simulink model "ParmTests"  (Simulink 7.5)
settings: Solver=ode45  StartTime=0.0  StopTime=10.0  RelTol=1e-3
settings Model: Creator=Robert  LastModifiedBy=Robert

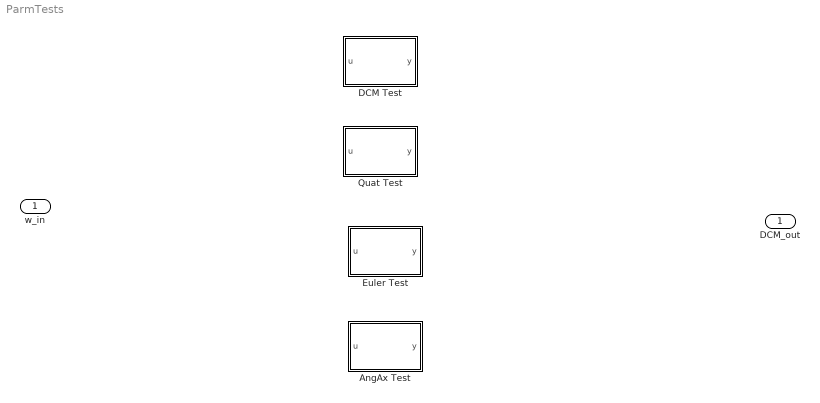
== system ParmTests ==
  w_in : Inport  OutDataType=fixdt(1, 16)  OutScaling=2^0
  AngAx Test : Stateflow chart  TreatAsAtomicUnit=on
  DCM Test : Stateflow chart  TreatAsAtomicUnit=on
  Euler Test : Stateflow chart  TreatAsAtomicUnit=on
  Quat Test : Stateflow chart  TreatAsAtomicUnit=on
  DCM_out : Outport  OutDataType=fixdt(1, 16)  OutScaling=2^0

== matlab function Quat Test ==
  data: u input double; y output double
function y = fcn(u)
%#eml

y = u;

== matlab function Euler Test ==
  data: u input double; y output double
function y = fcn(u)
%#eml

y = u;

== matlab function AngAx Test ==
  data: u input double; y output double
function y = fcn(u)
%#eml

y = u;

== matlab function DCM Test ==
  data: u input double; y output double
function y = fcn(u)
%#eml

y = u;
